simulink model "model32slx"  (R2024a)
settings: Solver=VariableStepAuto  StartTime=0.0  StopTime=10.0  MaxStep=1e-4  RelTol=1e-4
values from neighbouring files (symbols this model uses):
  A = [8 1 11 ... (first row only)    [init.m]    (also in init_ex.m)
  B = [-1; -3; 3]    [init.m]    (also in init_ex.m)
  B_f = [1, -1 ... (first row only)    [init.m]    (also in init_ex.m)
  C = [-2 0 -3]    [init.m]    (also in init_ex.m)
  D = 15    [init.m]    (also in init_ex.m)
  D_f = [0 3]    [init.m]    (also in init_ex.m)
  G = [-5 0 0 ... (first row only)    [init.m]    (also in init_ex.m)
  G_ex = diag([-1, -2, -3, -4])    [init_ex.m]
  G_f = [35 10 -28 17 ... (first row only)    [init.m]    (also in init_ex.m)
  G_g = [0 0 0 ... (first row only)    [init.m]    (also in init_ex.m)
  K = [-3.5 1 -3.5]    [init.m]    (also in init_ex.m)
  K_f = [-9.2262   -2.9556    6.9958   -4.9150]    [init.m]    (also in init_ex.m)
  K_g = [0.0703   -0.0562    0.0658]    [init.m]    (also in init_ex.m)
  Q_inv = inv(Q)    [init.m]    (also in init_ex.m)
  Qinv_ex = inv(Q_ex)    [init_ex.m]
  wf0 = [1; 1; 1; 1]    [init.m]    (also in init_ex.m)
  wg0 = [-12; 0; 21]    [init.m]    (also in init_ex.m)
  x0 = [0; 0; 0]    [init.m]    (also in init_ex.m)
  Y = [1; 7; 8]    [init.m]    (also in init_ex.m)
  Y_ex = [1; 1; 1; 1]    [init_ex.m]
  Y_f = [12 -6 ... (first row only)    [init.m]    (also in init_ex.m)
  Y_g = [1, 1, 0]    [init.m]    (also in init_ex.m)
settings Model: Creator=eva  LastModifiedBy=eva

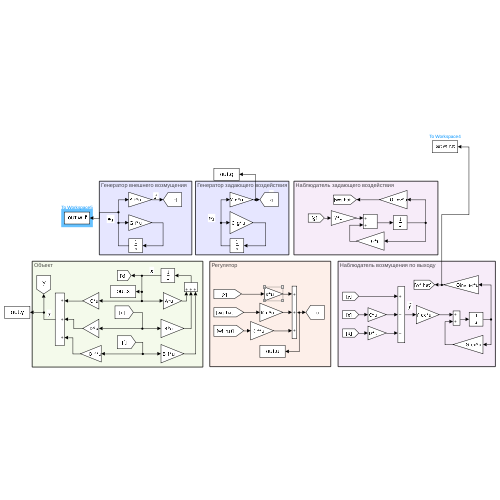
[thumbnail: Simulink's stored preview of the top-level diagram]
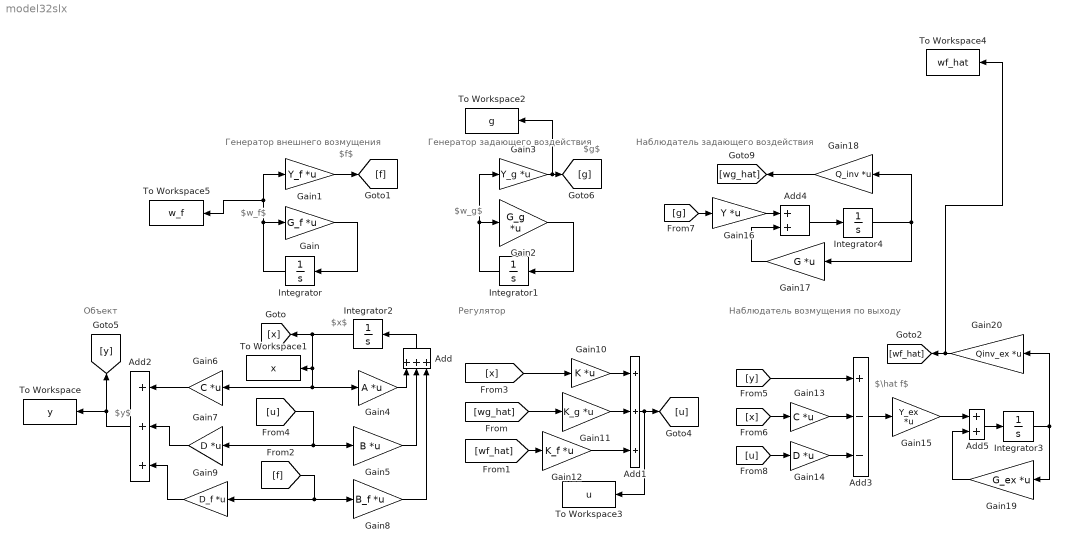
== system model32slx ==
  note: Генератор задающего воздействия
  note: $g$
  note: $w_g$
  note: $w_f$
  note: Наблюдатель возмущения по выходу
  note: $f$
  note: $x$
  note: Наблюдатель задающего воздействия
  note: Регулятор
  note: Генератор внешнего возмущения
  note: Объект
  note: $y$
  note: $\hat f$
  Add : Sum  Inputs=+++
  Add1 : Sum  Inputs=+++
  Add2 : Sum  Inputs=+++
  Add3 : Sum  Inputs=+--
  Add4 : Sum
  Add5 : Sum
  Gain : Gain  Gain=G_f  Multiplication=Matrix(K*u)
  Gain1 : Gain  Gain=Y_f  Multiplication=Matrix(K*u)
  Gain10 : Gain  Gain=K  Multiplication=Matrix(K*u)
  Gain11 : Gain  Gain=K_g  Multiplication=Matrix(K*u)
  Gain12 : Gain  Gain=K_f  Multiplication=Matrix(K*u)
  Gain13 : Gain  Gain=C  Multiplication=Matrix(K*u)
  Gain14 : Gain  Gain=D  Multiplication=Matrix(K*u)
  Gain15 : Gain  Gain=Y_ex  Multiplication=Matrix(K*u)
  Gain16 : Gain  Gain=Y  Multiplication=Matrix(K*u)
  Gain17 : Gain  Gain=G  Multiplication=Matrix(K*u)
  Gain18 : Gain  Gain=Q_inv  Multiplication=Matrix(K*u)
  Gain19 : Gain  Gain=G_ex  Multiplication=Matrix(K*u)
  Gain2 : Gain  Gain=G_g  Multiplication=Matrix(K*u)
  Gain20 : Gain  Gain=Qinv_ex  Multiplication=Matrix(K*u)
  Gain3 : Gain  Gain=Y_g  Multiplication=Matrix(K*u)
  Gain4 : Gain  Gain=A  Multiplication=Matrix(K*u)
  Gain5 : Gain  Gain=B  Multiplication=Matrix(K*u)
  Gain6 : Gain  Gain=C  Multiplication=Matrix(K*u)
  Gain7 : Gain  Gain=D  Multiplication=Matrix(K*u)
  Gain8 : Gain  Gain=B_f  Multiplication=Matrix(K*u)
  Gain9 : Gain  Gain=D_f  Multiplication=Matrix(K*u)
  Integrator : Integrator  InitialCondition=wf0
  Integrator1 : Integrator  InitialCondition=wg0
  Integrator2 : Integrator  InitialCondition=x0
  Integrator3 : Integrator
  Integrator4 : Integrator  InitialCondition=[0; 0; 0]
  To Workspace : ToWorkspace  VariableName=y  SaveFormat=Structure With Time  SampleTime=-1
  To Workspace1 : ToWorkspace  VariableName=x  SaveFormat=Structure With Time  SampleTime=-1
  To Workspace2 : ToWorkspace  VariableName=g  SaveFormat=Structure With Time  SampleTime=-1
  To Workspace3 : ToWorkspace  VariableName=u  SaveFormat=Structure With Time  SampleTime=-1
  To Workspace4 : ToWorkspace  VariableName=wf_hat  SaveFormat=Structure With Time  SampleTime=-1
  To Workspace5 : ToWorkspace  VariableName=w_f  SaveFormat=Structure With Time  SampleTime=-1
  wires:
  Gain2/1 -> Integrator1/1
  [x] -> Gain10/1
  Integrator/1 -> Gain/1, To Workspace5/1, Gain1/1
  Gain7/1 -> Add2/2
  Add2/1 -> [y], To Workspace/1
  Add/1 -> Integrator2/1
  Gain4/1 -> Add/1
  Gain11/1 -> Add1/2
  Gain9/1 -> Add2/3
  Gain10/1 -> Add1/1
  Gain17/1 -> Add4/2
  Gain6/1 -> Add2/1
  Integrator1/1 -> Gain2/1, Gain3/1
  Integrator2/1 -> To Workspace1/1, Gain6/1, Gain4/1, [x]
  Gain18/1 -> [wg_hat]
  Add4/1 -> Integrator4/1
  Gain8/1 -> Add/3
  Gain5/1 -> Add/2
  Integrator4/1 -> Gain17/1, Gain18/1
  Add1/1 -> To Workspace3/1, [u]
  [wf_hat] -> Gain12/1
  [u] -> Gain7/1, Gain5/1
  [wg_hat] -> Gain11/1
  Gain3/1 -> To Workspace2/1, [g]
  [f] -> Gain8/1, Gain9/1
  Gain12/1 -> Add1/3
  [g] -> Gain16/1
  Gain/1 -> Integrator/1
  Gain1/1 -> [f]
  Gain16/1 -> Add4/1
  [u] -> Gain14/1
  [x] -> Gain13/1
  Gain14/1 -> Add3/3
  Gain13/1 -> Add3/2
  [y] -> Add3/1
  Add3/1 -> Gain15/1
  Gain15/1 -> Add5/1
  Add5/1 -> Integrator3/1
  Gain19/1 -> Add5/2
  Integrator3/1 -> Gain20/1, Gain19/1
  Gain20/1 -> To Workspace4/1, [wf_hat]
